simulink subsystem "PieroenBC"  (R2023b)
settings: Solver=VariableStepAuto  StartTime=0.0  StopTime=10.0  RelTol=1e-3
settings Model: Creator=Usuario_UMA  LastModifiedBy=Usuario_UMA

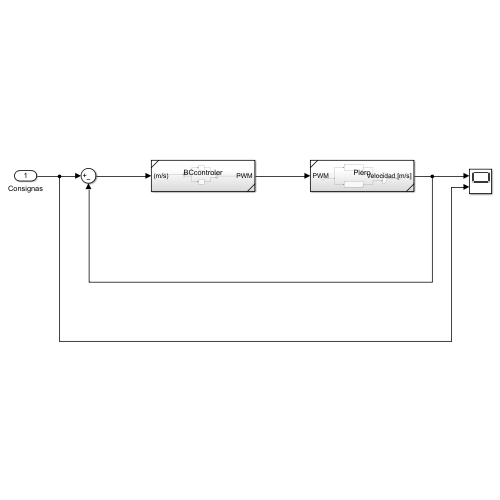
[thumbnail: Simulink's stored preview of the top-level diagram]
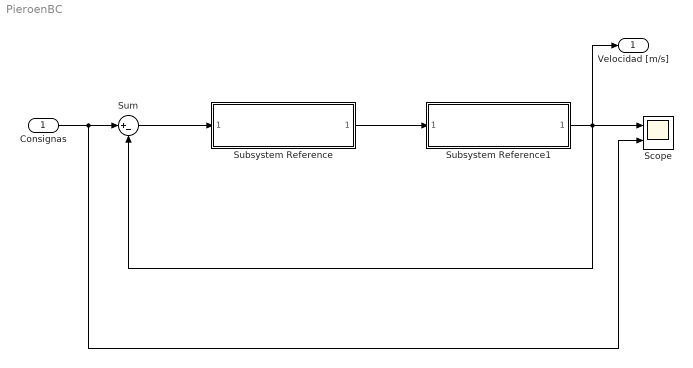
== system PieroenBC ==
  Consignas : Inport
  Scope : Scope  NumInputPorts=2
  Subsystem Reference : Subsystem  ReferencedSubsystem=BCcontroler
  Subsystem Reference1 : Subsystem  ReferencedSubsystem=Piero
  Sum : Sum  Inputs=|+-
  Velocidad [m/s] : Outport
  wires:
  Subsystem Reference1/1 -> Scope/1, Sum/2, Velocidad [m/s]/1
  Consignas/1 -> Scope/2, Sum/1
  Subsystem Reference/1 -> Subsystem Reference1/1
  Sum/1 -> Subsystem Reference/1
